simulink subsystem "CycleDetector"  (R2024b)
settings: Solver=VariableStepAuto  StartTime=0.0  StopTime=10.0  RelTol=1e-3
undefined symbols (not defined in the file or in its folder): DiscIntNeverNeededParam
libraries: simulink x1, dspsigops x1
settings Model: Creator=JesseJabezArendse  LastModifiedBy=JesseJabezArendse
settings RTWCC: GPUComputeCapability=3.5

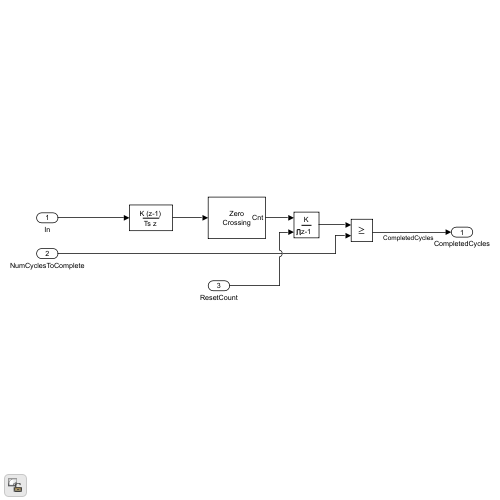
[thumbnail: Simulink's stored preview of the top-level diagram]
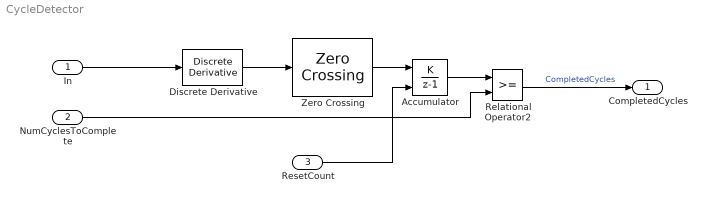
== system CycleDetector ==
  In : Inport
  NumCyclesToComplete : Inport  Port=2
  ResetCount : Inport  Port=3
  Accumulator : DiscreteIntegrator  IntegratorMethod=Accumulation: Forward Euler  ExternalReset=level  SampleTime=-1  OutDataTypeStr=Inherit: Inherit via back propagation  ICPrevOutput=DiscIntNeverNeededParam  ICPrevScaledInput=DiscIntNeverNeededParam
  Discrete Derivative : simulink/Discrete/Discrete Derivative  gainval=1.0  ICPrevScaledInput=0.0  OutMin=[]  OutMax=[]  OutDataType=fixdt(1, 16)  OutScaling=2^-10  DoSatur=off
  Relational Operator2 : RelationalOperator  RndMeth=Simplest  InputSameDT=off
  Zero Crossing : dspsigops/Zero Crossing
  CompletedCycles : Outport
  wires:
  Zero Crossing/1 -> Accumulator/1
  In/1 -> Discrete Derivative/1
  ResetCount/1 -> Accumulator/2
  Discrete Derivative/1 -> Zero Crossing/1
  Accumulator/1 -> Relational Operator2/1
  Relational Operator2/1 -> CompletedCycles/1  "CompletedCycles"
  NumCyclesToComplete/1 -> Relational Operator2/2
